simulink model "CTRL_SPECCTRL_FB_STRAT1_test"  (R2024b)
settings: Solver=VariableStepAuto  StartTime=0.0  StopTime=10.0  RelTol=1e-3
libraries: CTRL_SPECCTRL_FB_STRAT1 x1
settings Model: Creator=blatak  LastModifiedBy=blatak

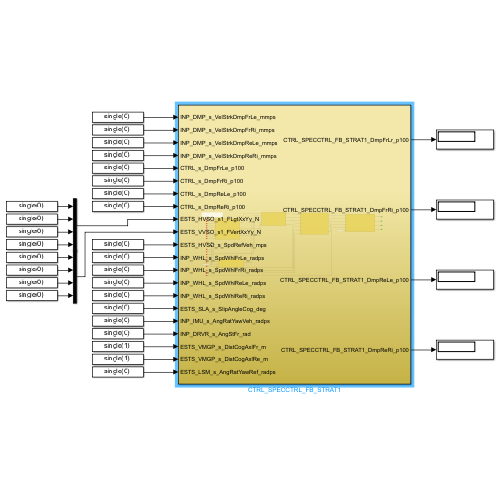
[thumbnail: Simulink's stored preview of the top-level diagram]
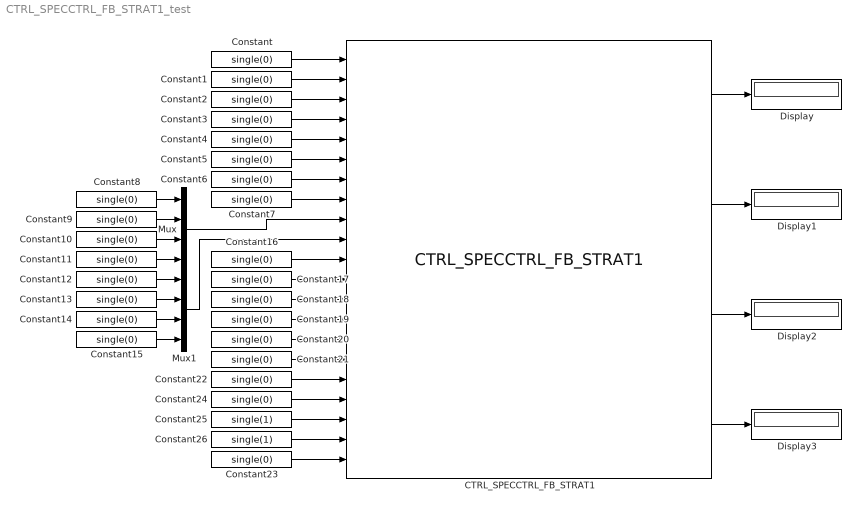
== system CTRL_SPECCTRL_FB_STRAT1_test ==
  CTRL_SPECCTRL_FB_STRAT1 : CTRL_SPECCTRL_FB_STRAT1/CTRL_SPECCTRL_FB_STRAT1  SystemSampleTime=-1  VariantActivationTime=update diagram  AllowFlexibleInterface=on  Latency=0  AutoFrameSizeCalculation=off
  Constant{,1..24} (25 alike) : Constant  Value=single(0)
  Constant25 : Constant  Value=single(1)
  Constant26 : Constant  Value=single(1)
  Display{,1..3} (4 alike) : Display
  Mux : Mux
  Mux1 : Mux
  wires:
  Constant18/1 -> CTRL_SPECCTRL_FB_STRAT1/13
  Constant23/1 -> CTRL_SPECCTRL_FB_STRAT1/21
  Constant26/1 -> CTRL_SPECCTRL_FB_STRAT1/20
  Constant25/1 -> CTRL_SPECCTRL_FB_STRAT1/19
  Constant24/1 -> CTRL_SPECCTRL_FB_STRAT1/18
  Constant22/1 -> CTRL_SPECCTRL_FB_STRAT1/17
  Constant21/1 -> CTRL_SPECCTRL_FB_STRAT1/16
  Constant20/1 -> CTRL_SPECCTRL_FB_STRAT1/15
  Constant19/1 -> CTRL_SPECCTRL_FB_STRAT1/14
  Constant17/1 -> CTRL_SPECCTRL_FB_STRAT1/12
  Constant16/1 -> CTRL_SPECCTRL_FB_STRAT1/11
  Constant8/1 -> Mux/1
  Constant9/1 -> Mux/2
  Constant10/1 -> Mux/3
  Constant11/1 -> Mux/4
  Constant12/1 -> Mux1/1
  Constant13/1 -> Mux1/2
  Constant14/1 -> Mux1/3
  Constant15/1 -> Mux1/4
  Constant/1 -> CTRL_SPECCTRL_FB_STRAT1/1
  Constant1/1 -> CTRL_SPECCTRL_FB_STRAT1/2
  Constant2/1 -> CTRL_SPECCTRL_FB_STRAT1/3
  Constant3/1 -> CTRL_SPECCTRL_FB_STRAT1/4
  Constant4/1 -> CTRL_SPECCTRL_FB_STRAT1/5
  Constant5/1 -> CTRL_SPECCTRL_FB_STRAT1/6
  Constant6/1 -> CTRL_SPECCTRL_FB_STRAT1/7
  Constant7/1 -> CTRL_SPECCTRL_FB_STRAT1/8
  Mux/1 -> CTRL_SPECCTRL_FB_STRAT1/9
  Mux1/1 -> CTRL_SPECCTRL_FB_STRAT1/10
  CTRL_SPECCTRL_FB_STRAT1/1 -> Display/1
  CTRL_SPECCTRL_FB_STRAT1/2 -> Display1/1
  CTRL_SPECCTRL_FB_STRAT1/3 -> Display2/1
  CTRL_SPECCTRL_FB_STRAT1/4 -> Display3/1
